simulink model "SWC_HALIN_CDD_type"  (R2021b)
settings: Solver=FixedStepDiscrete  StartTime=0.0  StopTime=10.0  FixedStep=0.005  RelTol=1e-3
undefined symbols (not defined in the file): C_TASK_5MS_S, DIDLen_APSFunConfig, DIDLen_AutoLock, DIDLen_AutoWipHSpdEN, DIDLen_DKCKey, DIDLen_DRLDis, DIDLen_DynoMode, DIDLen_FMHTimer, DIDLen_OBDReq, DIDLen_TestGroup, DIDLen_TireSize, DIDLen_USSConfig, DIDLen_WipRLSCmdCutFilter, DIDLen_WipRLSCmdHoldFilter, DIDLen_XWDMode, DIDNum_APSFunConfig, DIDNum_AutoLock, DIDNum_AutoWipHSpdEN, DIDNum_DKCKey, DIDNum_DRLDis, DIDNum_DynoMode, DIDNum_FMHTimer, DIDNum_OBDReq, DIDNum_TestGroup, DIDNum_TireSize, DIDNum_USSConfig, DIDNum_WipRLSCmdCutFilter, DIDNum_WipRLSCmdHoldFilter, DIDNum_XWDMode, ENUM_DRIVETRAIN_AWD, ENUM_DRIVETRAIN_FWD, ENUM_DRIVETRAIN_RWD, ENUM_REGENLEVEL_LV1, ENUM_REGENLEVEL_LV2, ENUM_REGENLEVEL_LV3, ENUM_REGENLEVEL_LV4, ENUM_REGENLEVEL_LV5, ENUM_REGENLEVEL_OPD, ENUM_TPMSSTA_FAT, ENUM_TPMSSTA_LOWBATTERY, ENUM_TPMSSTA_TRIGGER, FALSE, FIVE_INT, FOUR_INT, KHAL_CANBusOffDebounce_s, KHAL_DefaultRegenMode_enum, KHAL_DKCDecryptEnable_flg_ovrdflg, KHAL_DKCDecryptEnable_flg_ovrdval, KHAL_RandomNumberY1_enum, KHAL_RandomNumberY2_enum, KHAL_RandomNumberY_ovrdflg, KHAL_TPMSRESBUTT_flg_ovrdflg, KHAL_TPMSRESBUTT_flg_ovrdval, KINP_ReadVinCode_flg, ONE_INT, SIX_INT, THREE_INT, TRUE, TWO_INT, ZERO_FLOAT ... (+1)
libraries: simulink x112, hcu_lib x21, hdlsllib x15, FVT_lib x2
(part 6 of 7)

== system SWC_HALIN_CDD_type/run_SWC_HALIN_CDD_Rx_5ms_sys/Halin_CDD/Halin_SYS/RemoteControlSignal ==
  DT_CAN5_SG_TBOX1 : Inport
  CbnPreACEnaReq : Subsystem
  DrvWdwCtrlCmd : Subsystem
  PasWdwCtrlCmd : Subsystem
  PowerOffTSet : Subsystem
  RLDWdwCtrlCmd : Subsystem
  RRDWdwCtrlCmd : Subsystem
  ReDoorLock : Subsystem
  ReOutsideMirror : Subsystem
  RePwrReqTbox : Subsystem
  ReRadio : Subsystem
  RemoteACTemp : Subsystem
  RemoteAutoReq : Subsystem
  TBOXRemotePW : Subsystem
  bus_selector : BusSelector  OutputSignals=CAN5_FDC_Conn_CbnPreACEnaReq
  bus_selector1 : BusSelector  OutputSignals=CAN5_FDC_Conn_PowerOff_T_Set
  bus_selector11 : BusSelector  OutputSignals=CAN5_FDC_Conn_DrvWdwCtrl_Cmd
  bus_selector12 : BusSelector  OutputSignals=CAN5_FDC_Conn_PasWdwCtrl_Cmd
  bus_selector13 : BusSelector  OutputSignals=CAN5_FDC_Conn_RLDWdwCtrl_Cmd
  bus_selector14 : BusSelector  OutputSignals=CAN5_FDC_Conn_RRDWdwCtrl_Cmd
  bus_selector2 : BusSelector  OutputSignals=CAN5_FDC_Conn_ReOutsideMirror
  bus_selector3 : BusSelector  OutputSignals=CAN5_FDC_Conn_Re_DoorLock
  bus_selector4 : BusSelector  OutputSignals=CAN5_FDC_Conn_Re_PwrReq
  bus_selector5 : BusSelector  OutputSignals=CAN5_FDC_Conn_Re_Radio
  bus_selector6 : BusSelector  OutputSignals=CAN5_FDC_Conn_Remote_ACTemp
  bus_selector7 : BusSelector  OutputSignals=CAN5_FDC_Conn_Remote_AutoReq
  bus_selector9 : BusSelector  OutputSignals=CAN5_FDC_Conn_Remote_PW
  VHAL_CbnPreACEnaReq_enum : Outport
  VHAL_PowerOffTSet_cnt : Outport  Port=2
  VHAL_ReOutsideMirror_enum : Outport  Port=3
  VHAL_ReDoorLock_enum : Outport  Port=4
  VHAL_RePwrReqTbox_enum : Outport  Port=5
  VHAL_ReRadio_flg : Outport  Port=6
  VHAL_RemoteACTemp_C : Outport  Port=7
  VHAL_RemoteAutoReq_flg : Outport  Port=8
  VHAL_TBOXRemotePW_enum : Outport  Port=9
  VHAL_FDCConnDrvWdwCtrlCmd_pct : Outport  Port=10
  VHAL_FDCConnPasWdwCtrlCmd_pct : Outport  Port=11
  VHAL_FDCConnRLDWdwCtrlCmd_pct : Outport  Port=12
  VHAL_FDCConnRRDWdwCtrlCmd_pct : Outport  Port=13
  wires:
  DT_CAN5_SG_TBOX1/1 -> [DT_CAN5_SG_TBOX1]
  [DT_CAN5_SG_TBOX1] -> bus_selector/1
  bus_selector/1 -> CbnPreACEnaReq/1(CbnPreACEnaReq)  "<CAN5_FDC_Conn_CbnPreACEnaReq>"
  CbnPreACEnaReq/1(VHAL_CbnPreACEnaReq_enum) -> VHAL_CbnPreACEnaReq_enum/1  "VHAL_CbnPreACEnaReq_enum"
  [DT_CAN5_SG_TBOX1] -> bus_selector1/1
  bus_selector1/1 -> PowerOffTSet/1(PowerOff_T_Set)  "<CAN5_FDC_Conn_PowerOff_T_Set>"
  PowerOffTSet/1(VHAL_PowerOffTSet_cnt) -> VHAL_PowerOffTSet_cnt/1  "VHAL_PowerOffTSet_cnt"
  [DT_CAN5_SG_TBOX1] -> bus_selector2/1
  bus_selector2/1 -> ReOutsideMirror/1(ReOutsideMirror)  "<CAN5_FDC_Conn_ReOutsideMirror>"
  ReOutsideMirror/1(VHAL_ReOutsideMirror_enum) -> VHAL_ReOutsideMirror_enum/1  "VHAL_ReOutsideMirror_enum"
  [DT_CAN5_SG_TBOX1] -> bus_selector3/1
  bus_selector3/1 -> ReDoorLock/1(Re_DoorLock)  "<CAN5_FDC_Conn_Re_DoorLock>"
  ReDoorLock/1(VHAL_ReDoorLock_enum) -> VHAL_ReDoorLock_enum/1  "VHAL_ReDoorLock_enum"
  [DT_CAN5_SG_TBOX1] -> bus_selector4/1
  bus_selector4/1 -> RePwrReqTbox/1(Re_PwrReqTbox)  "<CAN5_FDC_Conn_Re_PwrReq>"
  RePwrReqTbox/1(VHAL_RePwrReqTbox_enum) -> VHAL_RePwrReqTbox_enum/1  "VHAL_RePwrReqTbox_enum"
  [DT_CAN5_SG_TBOX1] -> bus_selector5/1
  bus_selector5/1 -> ReRadio/1(Re_Radio)  "<CAN5_FDC_Conn_Re_Radio>"
  ReRadio/1(VHAL_ReRadio_flg) -> VHAL_ReRadio_flg/1  "VHAL_ReRadio_flg"
  [DT_CAN5_SG_TBOX1] -> bus_selector6/1
  bus_selector6/1 -> RemoteACTemp/1(Remote_ACTemp)  "<CAN5_FDC_Conn_Remote_ACTemp>"
  RemoteACTemp/1(VHAL_RemoteACTemp_C) -> VHAL_RemoteACTemp_C/1  "VHAL_RemoteACTemp_C"
  [DT_CAN5_SG_TBOX1] -> bus_selector7/1
  bus_selector7/1 -> RemoteAutoReq/1(Remote_AutoReq)  "<CAN5_FDC_Conn_Remote_AutoReq>"
  RemoteAutoReq/1(VHAL_RemoteAutoReq_flg) -> VHAL_RemoteAutoReq_flg/1  "VHAL_RemoteAutoReq_flg"
  [DT_CAN5_SG_TBOX1] -> bus_selector9/1
  bus_selector9/1 -> TBOXRemotePW/1(TBOX_Remote_PW)  "<CAN5_FDC_Conn_Remote_PW>"
  TBOXRemotePW/1(VHAL_TBOXRemotePW_enum) -> VHAL_TBOXRemotePW_enum/1  "VHAL_TBOXRemotePW_enum"
  [DT_CAN5_SG_TBOX1] -> bus_selector11/1
  [DT_CAN5_SG_TBOX1] -> bus_selector12/1
  [DT_CAN5_SG_TBOX1] -> bus_selector13/1
  [DT_CAN5_SG_TBOX1] -> bus_selector14/1
  bus_selector11/1 -> DrvWdwCtrlCmd/1(<CAN5_FDC_Conn_DrvWdwCtrl_Cmd>)  "<CAN5_FDC_Conn_DrvWdwCtrl_Cmd>"
  DrvWdwCtrlCmd/1(Out1) -> VHAL_FDCConnDrvWdwCtrlCmd_pct/1  "VHAL_FDCConnDrvWdwCtrlCmd_pct"
  bus_selector12/1 -> PasWdwCtrlCmd/1(<CAN5_FDC_Conn_PasWdwCtrl_Cmd>)  "<CAN5_FDC_Conn_PasWdwCtrl_Cmd>"
  PasWdwCtrlCmd/1(Out1) -> VHAL_FDCConnPasWdwCtrlCmd_pct/1  "VHAL_FDCConnPasWdwCtrlCmd_pct"
  bus_selector13/1 -> RLDWdwCtrlCmd/1(<CAN5_FDC_Conn_RLDWdwCtrl_Cmd>)  "<CAN5_FDC_Conn_RLDWdwCtrl_Cmd>"
  RLDWdwCtrlCmd/1(Out1) -> VHAL_FDCConnRLDWdwCtrlCmd_pct/1  "VHAL_FDCConnRLDWdwCtrlCmd_pct"
  bus_selector14/1 -> RRDWdwCtrlCmd/1(<CAN5_FDC_Conn_RRDWdwCtrl_Cmd>)  "<CAN5_FDC_Conn_RRDWdwCtrl_Cmd>"
  RRDWdwCtrlCmd/1(Out1) -> VHAL_FDCConnRRDWdwCtrlCmd_pct/1  "VHAL_FDCConnRRDWdwCtrlCmd_pct"

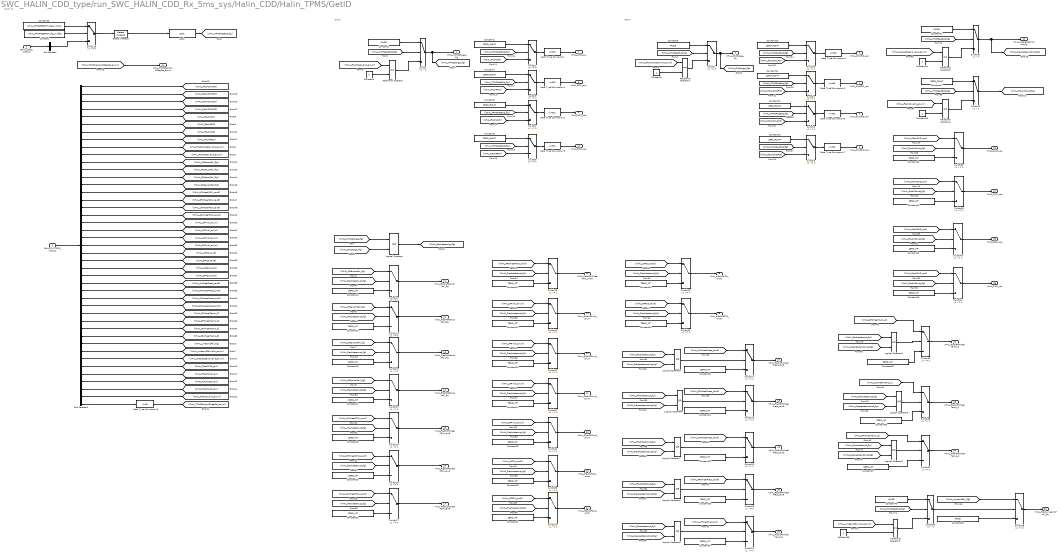
== system SWC_HALIN_CDD_type/run_SWC_HALIN_CDD_Rx_5ms_sys/Halin_CDD/Halin_TPMS/GetID ==
  note: FLASH ID
  note: GetID
  note: GetID
  BHAL_CAN2_outputs : Inport
  BHAL_SYSTPMS_outputs : Inport  Port=2
  Bus Selector : BusSelector  OutputSignals=VHAL_TPMSResButt_flg
  Bus Selector1 : BusSelector  OutputSignals=VHAL_FlashChkLFID_raw,VHAL_FlashChkRFID_raw,VHAL_FlashChkLRID_raw,VHAL_FlashChkRRID_raw,VHAL_FlashLFID_raw,VHAL_FlashRFID_raw,VHAL_FlashLRID_raw,VHAL_FlashRRID_raw,VHAL_Flashchkdatavalid_enum,VHAL_Flashdatavalid_enum,VHAL_LFSensorFail_flg,VHAL_RFSensorFail_flg,VHAL_LRSensorFail_flg,VHAL_RRSensorFail_flg,VHAL_LFWheelPSW_raw8,VHAL_RFWheelPSW_raw8,VHAL_LRWheelPSW_raw8,VHAL_RRWheelPSW_raw8,VHAL_LFPindi_enum,VHAL_RFPindi_enum,VHAL_LRPindi_enum,VHAL_RRPindi_enum,VHAL_LFP20_raw8,VHAL_RFP20_raw8,VHAL_LRP20_raw8,VHAL_RRP20_raw8,VHAL_LFWheelPress_raw8,VHAL_RFWheelPress_raw8,VHAL_LRWheelPress_raw8,VHAL_RRWheelPress_raw8,VHAL_LFWheelTemp_C,VHAL_RFWheelTemp_C,VHAL_LRWheelTemp_C,VHAL_RRWheelTemp_C,VHAL_unlearnSfali_flg,VHAL_unlearnSfailvalid_enum,VHAL_Prepresstempvalid_enum,VHAL_FlashS1ID_raw,VHAL_FlashS2ID_raw,VHAL_FlashS3ID_raw,VHAL_FlashS4ID_raw,VHAL_FlashIDvalid_enum,VHAL_TPMSSensorIDRegSta_raw
  Constant : Constant  Value=KHAL_TPMSRESBUTT_flg_ovrdflg
  Constant{1,7..13,47} (9 alike) : Constant  Value=ZERO_FLOAT
  Constant{14..37,43..46} (28 alike) : Constant  Value=ZERO_INT
  Constant{2..3,38,40..41} (5 alike) : Constant  Value=FALSE
  Constant{4..5,39,42,48} (5 alike) : Constant
  Constant6 : Constant  Value=KHAL_TPMSRESBUTT_flg_ovrdval
  Data Type Conversion{,1..7} (8 alike) : DataTypeConversion  OutDataTypeStr=uint32
  Data Type Conversion8 : DataTypeConversion  OutDataTypeStr=uint8
  Detect Increase : simulink/Logic and Bit Operations/Detect Increase  vinit=0.0  OutDataTypeStr=boolean
  Latch : hcu_lib/Basic_Blocks/Latch
  Logical Operator{,2..9} (9 alike) : Logic  Operator=OR  AllPortsSameDT=off  OutDataTypeStr=boolean
  Relational Operator{,1..4} (5 alike) : RelationalOperator  Operator===  OutDataTypeStr=boolean  RndMeth=Simplest
  Switch{,36..37,42} (4 alike) : Switch  Criteria=u2 > Threshold
  Switch{1..35,38..41} (39 alike) : Switch  Criteria=u2 ~= 0
  VHAL_TPMSStorge_flg : Outport
  VHAL_ChkStorge_flg : Outport  Port=2
  VHAL_ChkLFID_raw : Outport  Port=3
  VHAL_ChkRFID_raw : Outport  Port=4
  VHAL_ChkLRID_raw : Outport  Port=5
  VHAL_ChkRRID_raw : Outport  Port=6
  VHAL_LFID_raw : Outport  Port=7
  VHAL_RFID_raw : Outport  Port=8
  VHAL_LRID_raw : Outport  Port=9
  VHAL_RRID_raw : Outport  Port=10
  VHAL_FlashLFSensorFail_flg : Outport  Port=11
  VHAL_FlashRFSensorFail_flg : Outport  Port=12
  VHAL_FlashLRSensorFail_flg : Outport  Port=13
  VHAL_FlashRRSensorFail_flg : Outport  Port=14
  VHAL_FlashLFWheelPSW_raw8 : Outport  Port=15
  VHAL_FlashRFWheelPSW_raw8 : Outport  Port=16
  VHAL_FlashLRWheelPSW_raw8 : Outport  Port=17
  VHAL_FlashRRWheelPSW_raw8 : Outport  Port=18
  VHAL_FlashLFPindi_enum : Outport  Port=19
  VHAL_FlashRFPindi_enum : Outport  Port=20
  VHAL_FlashLRPindi_enum : Outport  Port=21
  VHAL_FlashRRPindi_enum : Outport  Port=22
  VHAL_FlashLFP20_raw8 : Outport  Port=23
  VHAL_FlashRFP20_raw8 : Outport  Port=24
  VHAL_FlashLRP20_raw8 : Outport  Port=25
  VHAL_FlashRRP20_raw8 : Outport  Port=26
  VHAL_FlashLFWheelPress_raw8 : Outport  Port=27
  VHAL_FlashRFWheelPress_raw8 : Outport  Port=28
  VHAL_FlashLRWheelPress_raw8 : Outport  Port=29
  VHAL_FlashRRWheelPress_raw8 : Outport  Port=30
  VHAL_FlashLFWheelTemp_C : Outport  Port=31
  VHAL_FlashRFWheelTemp_C : Outport  Port=32
  VHAL_FlashLRWheelTemp_C : Outport  Port=33
  VHAL_FlashRRWheelTemp_C : Outport  Port=34
  VHAL_FlashunlearnSfali_flg : Outport  Port=35
  VHAL_S1ID_raw : Outport  Port=36
  VHAL_S2ID_raw : Outport  Port=37
  VHAL_S3ID_raw : Outport  Port=38
  VHAL_S4ID_raw : Outport  Port=39
  VHAL_Prepresstemptrust_flg : Outport  Port=40
  VHAL_TPMSSensorIDRegSta_enum : Outport  Port=41
  wires:
  BHAL_CAN2_outputs/1 -> Bus Selector/1
  Latch/1 -> [VHAL_TPMSResButt_flg]
  [VHAL_TPMSResButt_flg] -> Switch4/2
  [VHAL_TPMSResButt_flg] -> Switch3/2
  [VHAL_FlashChkLFID] -> Switch6/3
  Switch3/1 -> Data Type Conversion1/1
  [VHAL_FlashRFID] -> Switch3/3
  Constant12/1 -> Switch8/1
  Constant9/1 -> Switch5/1
  [VHAL_FlashRRID] -> Switch5/3
  Constant1/1 -> Switch2/1
  Constant7/1 -> Switch3/1
  [VHAL_TPMSResButt_flg] -> Switch9/2
  [VHAL_TPMSResButt_flg] -> Switch2/2
  [VHAL_FlashLRID] -> Switch4/3
  Constant8/1 -> Switch4/1
  Switch2/1 -> Data Type Conversion/1
  [VHAL_TPMSResButt_flg] -> Switch5/2
  Switch4/1 -> Data Type Conversion2/1
  [VHAL_FlashChkLRID] -> Switch8/3
  [VHAL_FlashChkRRID] -> Switch9/3
  Constant10/1 -> Switch6/1
  Constant11/1 -> Switch7/1
  Switch8/1 -> Data Type Conversion6/1
  [VHAL_TPMSResButt_flg] -> Switch6/2
  Switch6/1 -> Data Type Conversion4/1
  Switch9/1 -> Data Type Conversion7/1
  Constant13/1 -> Switch9/1
  Switch7/1 -> Data Type Conversion5/1
  [VHAL_TPMSResButt_flg] -> Switch8/2
  [VHAL_TPMSResButt_flg] -> Switch7/2
  Switch5/1 -> Data Type Conversion3/1
  [VHAL_FlashChkRFID] -> Switch7/3
  [VHAL_FlashLFID] -> Switch2/3
  Switch10/1 -> Detect Increase/1
  Constant/1 -> Switch10/2
  Constant6/1 -> Switch10/1
  Bus Selector/1 -> Switch10/3  "<VHAL_TPMSResButt_flg>"
  [VHAL_TPMSResButt_flg] -> Switch/2
  Switch/1 -> [VHAL_TPMSStorge_flg], VHAL_TPMSStorge_flg/1
  Constant2/1 -> Switch/1
  Constant3/1 -> Switch1/1
  Switch1/1 -> [VHAL_ChkStorge_flg], VHAL_ChkStorge_flg/1
  [VHAL_TPMSResButt_flg] -> Switch1/2
  [VHAL_Flashdatavalid_enum] -> Relational Operator/1
  Relational Operator/1 -> Switch/3
  Constant4/1 -> Relational Operator/2
  Constant5/1 -> Relational Operator1/2
  Relational Operator1/1 -> Switch1/3
  [VHAL_Flashchkdatavalid_enum] -> Relational Operator1/1
  [VHAL_TPMSStorge_flg] -> Logical Operator/1
  [VHAL_ChkStorge_flg] -> Logical Operator/2
  Logical Operator/1 -> [VHAL_Flashdatatrust_flg]
  [VHAL_Flashdatatrust_flg] -> Switch11/2
  [VHAL_LFSensorFail_flg] -> Switch11/1
  Constant14/1 -> Switch11/3
  Switch11/1 -> VHAL_FlashLFSensorFail_flg/1
  Constant15/1 -> Switch12/3
  [VHAL_Flashdatatrust_flg] -> Switch12/2
  Constant16/1 -> Switch13/3
  [VHAL_Flashdatatrust_flg] -> Switch13/2
  Constant17/1 -> Switch14/3
  [VHAL_Flashdatatrust_flg] -> Switch14/2
  Constant18/1 -> Switch15/3
  [VHAL_Flashdatatrust_flg] -> Switch15/2
  Constant19/1 -> Switch16/3
  [VHAL_Flashdatatrust_flg] -> Switch16/2
  Constant20/1 -> Switch17/3
  [VHAL_Flashdatatrust_flg] -> Switch17/2
  Constant21/1 -> Switch18/3
  [VHAL_Flashdatatrust_flg] -> Switch18/2
  [VHAL_RFSensorFail_flg] -> Switch12/1
  [VHAL_LRSensorFail_flg] -> Switch13/1
  [VHAL_RRSensorFail_flg] -> Switch14/1
  [VHAL_LFWheelPSW_raw8] -> Switch15/1
  [VHAL_RFWheelPSW_raw8] -> Switch16/1
  [VHAL_LRWheelPSW_raw8] -> Switch17/1
  [VHAL_RRWheelPSW_raw8] -> Switch18/1
  Constant22/1 -> Switch19/3
  [VHAL_Flashdatatrust_flg] -> Switch19/2
  Constant23/1 -> Switch20/3
  [VHAL_Flashdatatrust_flg] -> Switch20/2
  Constant24/1 -> Switch21/3
  [VHAL_Flashdatatrust_flg] -> Switch21/2
  Constant25/1 -> Switch22/3
  [VHAL_Flashdatatrust_flg] -> Switch22/2
  [VHAL_LFPindi_enum] -> Switch19/1
  [VHAL_RFPindi_enum] -> Switch20/1
  [VHAL_LRPindi_enum] -> Switch21/1
  [VHAL_RRPindi_enum] -> Switch22/1
  Constant26/1 -> Switch23/3
  [VHAL_Flashdatatrust_flg] -> Switch23/2
  [VHAL_LFP20_raw8] -> Switch23/1
  Constant27/1 -> Switch24/3
  [VHAL_Flashdatatrust_flg] -> Switch24/2
  [VHAL_RFP20_raw8] -> Switch24/1
  Constant28/1 -> Switch25/3
  [VHAL_Flashdatatrust_flg] -> Switch25/2
  [VHAL_LRP20_raw8] -> Switch25/1
  Constant29/1 -> Switch26/3
  [VHAL_Flashdatatrust_flg] -> Switch26/2
  [VHAL_RRP20_raw8] -> Switch26/1
  Constant30/1 -> Switch27/3
  [VHAL_LFWheelPress_raw8] -> Switch27/1
  Constant31/1 -> Switch28/3
  [VHAL_RFWheelPress_raw8] -> Switch28/1
  Constant32/1 -> Switch29/3
  [VHAL_LRWheelPress_raw8] -> Switch29/1
  Constant33/1 -> Switch30/3
  [VHAL_RRWheelPress_raw8] -> Switch30/1
  Constant34/1 -> Switch31/3
  [VHAL_LFWheelTemp_C] -> Switch31/1
  Constant35/1 -> Switch32/3
  [VHAL_RFWheelTemp_C] -> Switch32/1
  Constant36/1 -> Switch33/3
  [VHAL_LRWheelTemp_C] -> Switch33/1
  Constant37/1 -> Switch34/3
  Logical Operator2/1 -> Switch34/2
  Constant38/1 -> Switch35/3
  [VHAL_unlearnSfali_flg] -> Switch35/1
  [VHAL_RRWheelTemp_C] -> Switch34/1
  Switch12/1 -> VHAL_FlashRFSensorFail_flg/1
  Switch13/1 -> VHAL_FlashLRSensorFail_flg/1
  Switch14/1 -> VHAL_FlashRRSensorFail_flg/1
  Switch15/1 -> VHAL_FlashLFWheelPSW_raw8/1
  Switch16/1 -> VHAL_FlashRFWheelPSW_raw8/1
  Switch17/1 -> VHAL_FlashLRWheelPSW_raw8/1
  Switch18/1 -> VHAL_FlashRRWheelPSW_raw8/1
  Switch19/1 -> VHAL_FlashLFPindi_enum/1
  Switch20/1 -> VHAL_FlashRFPindi_enum/1
  Switch21/1 -> VHAL_FlashLRPindi_enum/1
  Switch22/1 -> VHAL_FlashRRPindi_enum/1
  Switch23/1 -> VHAL_FlashLFP20_raw8/1
  Switch24/1 -> VHAL_FlashRFP20_raw8/1
  Switch25/1 -> VHAL_FlashLRP20_raw8/1
  Switch26/1 -> VHAL_FlashRRP20_raw8/1
  Switch27/1 -> VHAL_FlashLFWheelPress_raw8/1
  Switch28/1 -> VHAL_FlashRFWheelPress_raw8/1
  Switch29/1 -> VHAL_FlashLRWheelPress_raw8/1
  Switch30/1 -> VHAL_FlashRRWheelPress_raw8/1
  Switch31/1 -> VHAL_FlashLFWheelTemp_C/1
  Switch32/1 -> VHAL_FlashRFWheelTemp_C/1
  Switch33/1 -> VHAL_FlashLRWheelTemp_C/1
  Switch34/1 -> VHAL_FlashRRWheelTemp_C/1
  [VHAL_unlearnSfailvalid_enum] -> Relational Operator2/1
  Constant39/1 -> Relational Operator2/2
  Constant40/1 -> Switch36/1
  [VHAL_TPMSResButt_flg] -> Switch36/2
  Switch35/1 -> VHAL_FlashunlearnSfali_flg/1
  Switch36/1 -> Switch35/2
  Relational Operator2/1 -> Switch36/3
  Constant42/1 -> Relational Operator3/2
  [VHAL_TPMSResButt_flg] -> Switch37/2
  Constant41/1 -> Switch37/1
  Relational Operator3/1 -> Switch37/3
  [VHAL_Prepresstempvalid_enum] -> Relational Operator3/1
  Switch37/1 -> VHAL_Prepresstemptrust_flg/1, [VHAL_Prepresstemptrust_flg]
  [VHAL_Flashdatatrust_flg] -> Logical Operator2/1
  [VHAL_Prepresstemptrust_flg] -> Logical Operator2/2
  [VHAL_Flashdatatrust_flg] -> Logical Operator3/1
  [VHAL_Prepresstemptrust_flg] -> Logical Operator3/2
  Logical Operator3/1 -> Switch33/2
  [VHAL_Flashdatatrust_flg] -> Logical Operator4/1
  [VHAL_Prepresstemptrust_flg] -> Logical Operator4/2
  Logical Operator4/1 -> Switch32/2
  [VHAL_Flashdatatrust_flg] -> Logical Operator5/1
  [VHAL_Prepresstemptrust_flg] -> Logical Operator5/2
  Logical Operator5/1 -> Switch31/2
  [VHAL_Flashdatatrust_flg] -> Logical Operator6/1
  [VHAL_Prepresstemptrust_flg] -> Logical Operator6/2
  Logical Operator6/1 -> Switch30/2
  [VHAL_Flashdatatrust_flg] -> Logical Operator7/1
  [VHAL_Prepresstemptrust_flg] -> Logical Operator7/2
  Logical Operator7/1 -> Switch29/2
  [VHAL_Flashdatatrust_flg] -> Logical Operator8/1
  [VHAL_Prepresstemptrust_flg] -> Logical Operator8/2
  Logical Operator8/1 -> Switch28/2
  [VHAL_Flashdatatrust_flg] -> Logical Operator9/1
  [VHAL_Prepresstemptrust_flg] -> Logical Operator9/2
  Logical Operator9/1 -> Switch27/2
  Detect Increase/1 -> Latch/1
  Data Type Conversion/1 -> VHAL_LFID_raw/1
  Data Type Conversion1/1 -> VHAL_RFID_raw/1
  Data Type Conversion2/1 -> VHAL_LRID_raw/1
  Data Type Conversion3/1 -> VHAL_RRID_raw/1
  Data Type Conversion4/1 -> VHAL_ChkLFID_raw/1
  Data Type Conversion5/1 -> VHAL_ChkRFID_raw/1
  Data Type Conversion6/1 -> VHAL_ChkLRID_raw/1
  Data Type Conversion7/1 -> VHAL_ChkRRID_raw/1
  Switch42/1 -> [VHAL_FlashIDtrust_flg]
  Constant45/1 -> Switch40/3
  Constant46/1 -> Switch41/3
  Constant44/1 -> Switch39/3
  Switch39/1 -> VHAL_S2ID_raw/1
  [VHAL_FlashS3ID_raw] -> Switch40/1
  [VHAL_FlashS2ID_raw] -> Switch39/1
  [VHAL_FlashS4ID_raw] -> Switch41/1
  Constant43/1 -> Switch38/3
  [VHAL_FlashS1ID_raw] -> Switch38/1
  [VHAL_TPMSResButt_flg] -> Switch42/2
  [VHAL_FlashIDtrust_flg] -> Switch38/2
  Switch41/1 -> VHAL_S4ID_raw/1
  [VHAL_FlashIDtrust_flg] -> Switch39/2
  Constant47/1 -> Switch42/1
  Switch40/1 -> VHAL_S3ID_raw/1
  Constant48/1 -> Relational Operator4/2
  [VHAL_FlashIDtrust_flg] -> Switch41/2
  Switch38/1 -> VHAL_S1ID_raw/1
  [VHAL_FlashIDvalid_enum] -> Relational Operator4/1
  Relational Operator4/1 -> Switch42/3
  [VHAL_FlashIDtrust_flg] -> Switch40/2
  Bus Selector1/35 -> [VHAL_unlearnSfali_flg]  "<VHAL_unlearnSfali_flg>"
  Bus Selector1/4 -> [VHAL_FlashChkRRID]  "<VHAL_FlashChkRRID_raw>"
  Bus Selector1/27 -> [VHAL_LFWheelPress_raw8]  "<VHAL_LFWheelPress_raw8>"
  Bus Selector1/19 -> [VHAL_LFPindi_enum]  "<VHAL_LFPindi_enum>"
  Bus Selector1/21 -> [VHAL_LRPindi_enum]  "<VHAL_LRPindi_enum>"
  Bus Selector1/25 -> [VHAL_LRP20_raw8]  "<VHAL_LRP20_raw8>"
  Bus Selector1/33 -> [VHAL_LRWheelTemp_C]  "<VHAL_LRWheelTemp_C>"
  Bus Selector1/26 -> [VHAL_RRP20_raw8]  "<VHAL_RRP20_raw8>"
  Bus Selector1/18 -> [VHAL_RRWheelPSW_raw8]  "<VHAL_RRWheelPSW_raw8>"
  Bus Selector1/32 -> [VHAL_RFWheelTemp_C]  "<VHAL_RFWheelTemp_C>"
  Bus Selector1/29 -> [VHAL_LRWheelPress_raw8]  "<VHAL_LRWheelPress_raw8>"
  Bus Selector1/8 -> [VHAL_FlashRRID]  "<VHAL_FlashRRID_raw>"
  Bus Selector1/12 -> [VHAL_RFSensorFail_flg]  "<VHAL_RFSensorFail_flg>"
  Bus Selector1/20 -> [VHAL_RFPindi_enum]  "<VHAL_RFPindi_enum>"
  Bus Selector1/11 -> [VHAL_LFSensorFail_flg]  "<VHAL_LFSensorFail_flg>"
  Bus Selector1/24 -> [VHAL_RFP20_raw8]  "<VHAL_RFP20_raw8>"
  Bus Selector1/22 -> [VHAL_RRPindi_enum]  "<VHAL_RRPindi_enum>"
  Bus Selector1/6 -> [VHAL_FlashRFID]  "<VHAL_FlashRFID_raw>"
  Bus Selector1/3 -> [VHAL_FlashChkLRID]  "<VHAL_FlashChkLRID_raw>"
  Bus Selector1/2 -> [VHAL_FlashChkRFID]  "<VHAL_FlashChkRFID_raw>"
  Bus Selector1/37 -> [VHAL_Prepresstempvalid_enum]  "<VHAL_Prepresstempvalid_enum>"
  Bus Selector1/34 -> [VHAL_RRWheelTemp_C]  "<VHAL_RRWheelTemp_C>"
  Bus Selector1/16 -> [VHAL_RFWheelPSW_raw8]  "<VHAL_RFWheelPSW_raw8>"
  Bus Selector1/30 -> [VHAL_RRWheelPress_raw8]  "<VHAL_RRWheelPress_raw8>"
  Bus Selector1/28 -> [VHAL_RFWheelPress_raw8]  "<VHAL_RFWheelPress_raw8>"
  Bus Selector1/14 -> [VHAL_RRSensorFail_flg]  "<VHAL_RRSensorFail_flg>"
  Bus Selector1/38 -> [VHAL_FlashS1ID_raw]  "<VHAL_FlashS1ID_raw>"
  Bus Selector1/41 -> [VHAL_FlashS4ID_raw]  "<VHAL_FlashS4ID_raw>"
  Bus Selector1/10 -> [VHAL_Flashdatavalid_enum]  "<VHAL_Flashdatavalid_enum>"
  Bus Selector1/15 -> [VHAL_LFWheelPSW_raw8]  "<VHAL_LFWheelPSW_raw8>"
  Bus Selector1/5 -> [VHAL_FlashLFID]  "<VHAL_FlashLFID_raw>"
  Bus Selector1/39 -> [VHAL_FlashS2ID_raw]  "<VHAL_FlashS2ID_raw>"
  BHAL_SYSTPMS_outputs/1 -> Bus Selector1/1
  Bus Selector1/9 -> [VHAL_Flashchkdatavalid_enum]  "<VHAL_Flashchkdatavalid_enum>"
  Bus Selector1/1 -> [VHAL_FlashChkLFID]  "<VHAL_FlashChkLFID_raw>"
  Bus Selector1/7 -> [VHAL_FlashLRID]  "<VHAL_FlashLRID_raw>"
  Bus Selector1/36 -> [VHAL_unlearnSfailvalid_enum]  "<VHAL_unlearnSfailvalid_enum>"
  Bus Selector1/23 -> [VHAL_LFP20_raw8]  "<VHAL_LFP20_raw8>"
  Bus Selector1/40 -> [VHAL_FlashS3ID_raw]  "<VHAL_FlashS3ID_raw>"
  Bus Selector1/13 -> [VHAL_LRSensorFail_flg]  "<VHAL_LRSensorFail_flg>"
  Bus Selector1/42 -> [VHAL_FlashIDvalid_enum]  "<VHAL_FlashIDvalid_enum>"
  Bus Selector1/31 -> [VHAL_LFWheelTemp_C]  "<VHAL_LFWheelTemp_C>"
  Bus Selector1/17 -> [VHAL_LRWheelPSW_raw8]  "<VHAL_LRWheelPSW_raw8>"
  Bus Selector1/43 -> Data Type Conversion8/1  "<VHAL_TPMSSensorIDRegSta_raw>"
  [VHAL_TPMSSensorIDRegSta_enum] -> VHAL_TPMSSensorIDRegSta_enum/1
  Data Type Conversion8/1 -> [VHAL_TPMSSensorIDRegSta_enum]  "VHAL_TPMSSensorIDRegSta_enum"

== system SWC_HALIN_CDD_type/run_SWC_HALIN_CDD_Rx_5ms_sys/Halin_CDD/Halin_TPMS/Subsystem ==
  note: Custom State Judgement
  note: Data Output
  note: Data Valid Judge
  TPMS_DataIn_flg : Inport
  TPMS_RawData : Inport  Port=2
  Add : Sum  Inputs=++++
  Bit Shift : hdlsllib/Logic and Bit Operations/Bit Shift  mode=Shift Left Logical  N=24
  Bit Shift1 : hdlsllib/Logic and Bit Operations/Bit Shift  mode=Shift Left Logical  N=16
  Bit Shift3 : hdlsllib/Logic and Bit Operations/Bit Shift  mode=Shift Left Logical  N=8
  Bitwise NOT : simulink/Logic and Bit Operations/Bitwise Operator  logicop=NOT  UseBitMask=off  BitMask=bin2dec('11011001')  BitMaskRealWorld=Stored Integer
  CRC8_Caculation : Subsystem
  Constant1 : Constant  Value=ENUM_TPMSSTA_TRIGGER
  Constant{4,7,9..10} (4 alike) : Constant  Value=TRUE
  Constant{5..6,8,11} (4 alike) : Constant  Value=FALSE
  Constant2 : Constant  Value=ENUM_TPMSSTA_LOWBATTERY
  Constant3 : Constant  Value=ENUM_TPMSSTA_FAT
  Data Type Conversion : DataTypeConversion  OutDataTypeStr=uint32
  Data Type Conversion1 : DataTypeConversion  OutDataTypeStr=uint8
  Data Type Conversion2 : DataTypeConversion  OutDataTypeStr=uint8
  Data Type Conversion3 : DataTypeConversion  OutDataTypeStr=uint32
  Data Type Conversion4 : DataTypeConversion  OutDataTypeStr=uint32
  Demux : Demux  Outputs=9
  Demux1 : Demux  Outputs=10
  Equal{,1..4} (5 alike) : RelationalOperator  Operator===  OutDataTypeStr=boolean  RndMeth=Simplest
  Logical Operator : Logic  Inputs=3  AllPortsSameDT=off  OutDataTypeStr=boolean
  Mux : Mux  Inputs=10
  Mux1 : Mux  Inputs=8
  Switch{,1..4} (5 alike) : Switch  Criteria=u2 ~= 0
  Unit Delay : UnitDelay  SampleTime=-1  HasFrameUpgradeWarning=on
  VHAL_TPMSDataIn_flg : Outport
  VHAL_TPMSID_raw : Outport  Port=2
  VHAL_TPMSPressure_raw : Outport  Port=3
  VHAL_TPMSTemp_raw : Outport  Port=4
  VHAL_TPMSSta_enum : Outport  Port=5
  VHAL_TPMSPressureMi_raw : Outport  Port=6
  VHAL_TPMSCRC_crc : Outport  Port=7
  VHAL_TPMSCRCCalc_crc : Outport  Port=8
  VHAL_TPMSFAT_flg : Outport  Port=9
  VHAL_TPMSBattLow_flg : Outport  Port=10
  VHAL_TPMSTrigger_flg : Outport  Port=11
  wires:
  TPMS_DataIn_flg/1 -> Data Type Conversion2/1
  [TPMSData] -> Demux/1
  Bit Shift/1 -> Add/1
  Bit Shift1/1 -> Add/2
  Bit Shift3/1 -> Add/3
  Add/1 -> VHAL_TPMSID_raw/1
  Demux/5 -> [Pressure]  "Pressure"
  Demux/7 -> [Status]  "Sta"
  Demux/8 -> [PressureMirror]  "PressureMirror"
  Demux/9 -> [CRC]  "CRC"
  Demux/1 -> [ID4]  "ID4"
  Demux/2 -> [ID3]  "ID3"
  Demux/3 -> [ID2]  "ID2"
  Demux/4 -> [ID1]  "ID1"
  Demux/6 -> [Temp]  "Temp"
  [Pressure] -> Bitwise NOT/1
  Bitwise NOT/1 -> Equal/1
  [PressureMirror] -> Equal/2
  [ID4] -> Mux1/1
  [ID3] -> Mux1/2
  [ID2] -> Mux1/3
  [ID1] -> Mux1/4
  [Pressure] -> Mux1/5
  [Temp] -> Mux1/6
  [Status] -> Mux1/7
  [PressureMirror] -> Mux1/8
  Mux1/1 -> CRC8_Caculation/1(MsgData)
  [CRC] -> Equal1/2
  Equal1/1 -> Logical Operator/1
  Equal/1 -> Logical Operator/2
  Logical Operator/1 -> [DataValid_flg]
  [DataValid_flg] -> Switch/2
  Mux/1 -> Switch/1
  Switch/1 -> Unit Delay/1, Demux1/1
  Unit Delay/1 -> Switch/3
  Data Type Conversion1/1 -> [TPMSData]
  Data Type Conversion2/1 -> [Data_in]
  CRC8_Caculation/1(CRCout) -> [CRC_Calc], Equal1/1  "CRC_Calc"
  Switch1/1 -> VHAL_TPMSFAT_flg/1
  [VHAL_TPMSSta_enum] -> Equal2/1
  Constant3/1 -> Equal2/2
  Equal2/1 -> Switch1/2
  Constant4/1 -> Switch1/1
  Constant5/1 -> Switch1/3
  Constant8/1 -> Switch2/3
  [VHAL_TPMSSta_enum] -> Equal3/1
  Constant7/1 -> Switch2/1
  Switch2/1 -> VHAL_TPMSBattLow_flg/1
  Equal3/1 -> Switch2/2
  Constant2/1 -> Equal3/2
  [Data_in] -> Logical Operator/3
  [DataValid_flg] -> Switch3/2
  Switch3/1 -> VHAL_TPMSDataIn_flg/1
  Constant6/1 -> Switch3/3
  Constant9/1 -> Switch3/1
  [ID4] -> Mux/1
  [ID3] -> Mux/2
  [ID2] -> Mux/3
  [ID1] -> Mux/4
  [Pressure] -> Mux/5
  [Temp] -> Mux/6
  [Status] -> Mux/7
  [PressureMirror] -> Mux/8
  [CRC] -> Mux/9
  [CRC_Calc] -> Mux/10
  Demux1/10 -> VHAL_TPMSCRCCalc_crc/1
  Demux1/9 -> VHAL_TPMSCRC_crc/1
  Demux1/8 -> VHAL_TPMSPressureMi_raw/1
  Demux1/7 -> [VHAL_TPMSSta_enum], VHAL_TPMSSta_enum/1
  Demux1/6 -> VHAL_TPMSTemp_raw/1
  Demux1/5 -> VHAL_TPMSPressure_raw/1
  Demux1/1 -> Data Type Conversion/1
  Demux1/2 -> Data Type Conversion3/1
  Demux1/3 -> Data Type Conversion4/1
  Data Type Conversion/1 -> Bit Shift/1
  Data Type Conversion3/1 -> Bit Shift1/1
  Data Type Conversion4/1 -> Bit Shift3/1
  Demux1/4 -> Add/4
  TPMS_RawData/1 -> Data Type Conversion1/1
  Equal4/1 -> Switch4/2
  Constant10/1 -> Switch4/1
  [VHAL_TPMSSta_enum] -> Equal4/1
  Constant11/1 -> Switch4/3
  Switch4/1 -> VHAL_TPMSTrigger_flg/1
  Constant1/1 -> Equal4/2

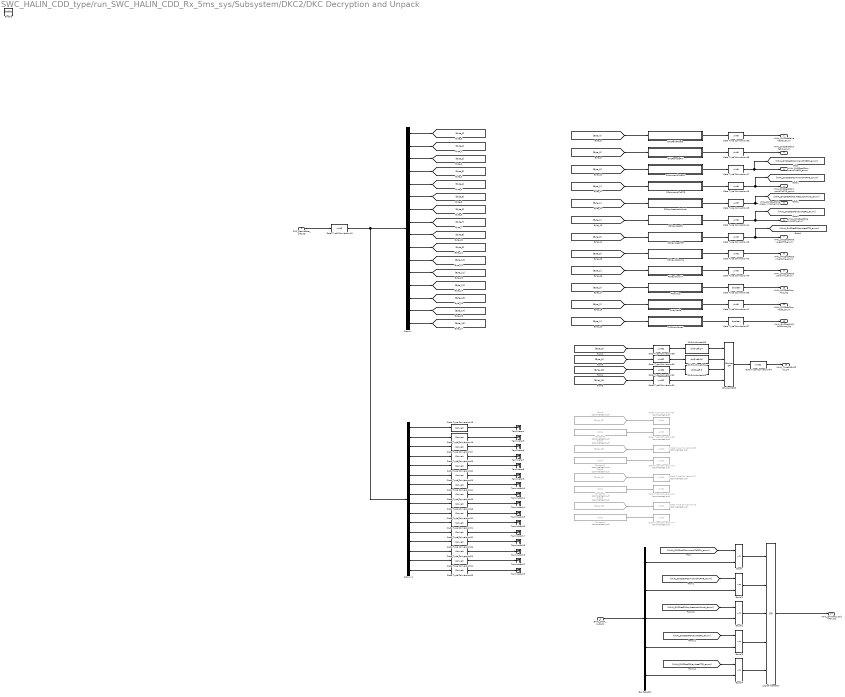
== system SWC_HALIN_CDD_type/run_SWC_HALIN_CDD_Rx_5ms_sys/Subsystem/DKC2/DKC Decryption and Unpack ==
  DKC_ResultData_16byte : Inport
  BHAL_CAN4_outputs : Inport  Port=2
  Enable : EnablePort
  Bitwise OR33 : simulink/Logic and Bit Operations/Bitwise Operator  logicop=OR  UseBitMask=off  NumInputPorts=4  BitMask=bin2dec('00000000000000000000')  BitMaskRealWorld=Stored Integer
  Bus Selector : BusSelector  OutputSignals=VHAL_PCommandToBCM_enum,VHAL_PCommandToPTG_enum,VHAL_PDKeyAreaLockUnlock_enum,VHAL_PDKeyAreaPS_enum,VHAL_PDKeyAreaPTG_enum
  Constant{1..4} (4 alike) : Constant  Commented=on  Value=0x04
  DKCReVehData : Subsystem  AncestorBlock=dkc2/DKC/Subsystem/VDKC_DKCDecryptionDATA_enum Unpack/DKCReVehData
  DKCRemotePW : Subsystem  AncestorBlock=dkc2/DKC/Subsystem/VDKC_DKCDecryptionDATA_enum Unpack/DKCRemotePW
  Data Type Conversion{16,38..47} (11 alike) : DataTypeConversion  OutDataTypeStr=uint8
  Data Type Conversion36 : DataTypeConversion  OutDataTypeStr=boolean
  Data Type Conversion37 : DataTypeConversion  OutDataTypeStr=boolean
  Data Type Conversion{48..57,59,62..66} (16 alike) : DataTypeConversion
  Data Type Conversion{58,60..61,81,94} (5 alike) : DataTypeConversion  OutDataTypeStr=uint32
  Data Type Conversion{67..74} (8 alike) : DataTypeConversion  Commented=on  OutDataTypeStr=uint8
  Demux : Demux  Outputs=16
  Demux1 : Demux  Outputs=16
  Equal{,1..4} (5 alike) : RelationalOperator  Operator=~=  OutDataTypeStr=boolean  RndMeth=Simplest
  From6 : From  Commented=on  GotoTag=Byte_12
  From7 : From  Commented=on  GotoTag=Byte_13
  From8 : From  Commented=on  GotoTag=Byte_14
  From9 : From  Commented=on  GotoTag=Byte_15
  Logical Operator : Logic  Operator=OR  Inputs=5  AllPortsSameDT=off  OutDataTypeStr=boolean
  PCommandToBCM : Subsystem  AncestorBlock=dkc2/DKC/Subsystem/VDKC_DKCDecryptionDATA_enum Unpack/PCommandToBCM
  PCommandToPTG : Subsystem  AncestorBlock=dkc2/DKC/Subsystem/VDKC_DKCDecryptionDATA_enum Unpack/PCommandToPTG
  PDKeyAreaLockUnlock : Subsystem  AncestorBlock=dkc2/DKC/Subsystem/VDKC_DKCDecryptionDATA_enum Unpack/PDKeyAreaLockUnlock
  PDKeyAreaPS : Subsystem  AncestorBlock=dkc2/DKC/Subsystem/VDKC_DKCDecryptionDATA_enum Unpack/PDKeyAreaPS
  PDKeyAreaPTG : Subsystem  AncestorBlock=dkc2/DKC/Subsystem/VDKC_DKCDecryptionDATA_enum Unpack/PDKeyAreaPTG
  PDKeyWelcome : Subsystem  AncestorBlock=dkc2/DKC/Subsystem/VDKC_DKCDecryptionDATA_enum Unpack/PDKeyWelcome
  PDkeyShowIVI : Subsystem  AncestorBlock=dkc2/DKC/Subsystem/VDKC_DKCDecryptionDATA_enum Unpack/PDkeyShowIVI
  PKeyMiss : Subsystem  AncestorBlock=dkc2/DKC/Subsystem/VDKC_DKCDecryptionDATA_enum Unpack/PKeyMiss
  PKeyMode : Subsystem  AncestorBlock=dkc2/DKC/Subsystem/VDKC_DKCDecryptionDATA_enum Unpack/PKeyMode
  PUIDLowPower : Subsystem  AncestorBlock=dkc2/DKC/Subsystem/VDKC_DKCDecryptionDATA_enum Unpack/PUIDLowPower
  Shift Arithmetic33 : ArithShift  BitShiftNumber=8  BitShiftDirection=Left
  Shift Arithmetic34 : ArithShift  BitShiftNumber=16  BitShiftDirection=Left
  Shift Arithmetic35 : ArithShift  BitShiftNumber=24  BitShiftDirection=Left
  Terminator{4..19} (16 alike) : Terminator
  VHAL_DKCDecReVehData_enum : Outport
  VHAL_DKCDecRemotePW_enum : Outport  Port=2
  VHAL_DKCDecPCommandToBCM_enum : Outport  Port=3
  VHAL_DKCDecPCommandToPTG_enum : Outport  Port=4
  VHAL_DKCDecPDKeyAreaLockUnlock_enum : Outport  Port=5
  VHAL_DKCDecPDKeyAreaPS_enum : Outport  Port=6
  VHAL_DKCDecPDKeyAreaPTG_enum : Outport  Port=7
  VHAL_DKCDecPDKeyWelcome_enum : Outport  Port=8
  VHAL_DKCDecPDkeyShowIVI_enum : Outport  Port=9
  VHAL_DKCDecPKeyMiss_flg : Outport  Port=10
  VHAL_DKCDecPKeyMode_enum : Outport  Port=11
  VHAL_DKCDecPUIDLowPower_flg : Outport  Port=12
  VHAL_TimeSNDKCFbk_cnt : Outport  Port=13
  VHAL_DKCDecryptionFail_flg : Outport  Port=14
  wires:
  Data Type Conversion53/1 -> Terminator19/1  "VHAL_DKCResultData_raw14"
  Demux1/6 -> Data Type Conversion63/1  "VHAL_DKCResultData_raw6"
  Demux1/16 -> Data Type Conversion55/1  "VHAL_DKCResultData_raw16"
  Data Type Conversion50/1 -> Terminator15/1  "VHAL_DKCResultData_raw10"
  Demux1/2 -> Data Type Conversion49/1  "VHAL_DKCResultData_raw2"
  Data Type Conversion62/1 -> Terminator8/1  "VHAL_DKCResultData_raw5"
  Data Type Conversion55/1 -> Terminator13/1  "VHAL_DKCResultData_raw16"
  Data Type Conversion49/1 -> Terminator5/1  "VHAL_DKCResultData_raw2"
  Data Type Conversion64/1 -> Terminator10/1  "VHAL_DKCResultData_raw7"
  Demux1/1 -> Data Type Conversion48/1  "VHAL_DKCResultData_raw1"
  Data Type Conversion48/1 -> Terminator4/1  "VHAL_DKCResultData_raw1"
  Data Type Conversion57/1 -> Terminator6/1  "VHAL_DKCResultData_raw3"
  Data Type Conversion56/1 -> Terminator18/1  "VHAL_DKCResultData_raw13"
  Demux1/14 -> Data Type Conversion53/1  "VHAL_DKCResultData_raw14"
  Demux1/10 -> Data Type Conversion50/1  "VHAL_DKCResultData_raw10"
  Demux1/7 -> Data Type Conversion64/1  "VHAL_DKCResultData_raw7"
  Demux1/8 -> Data Type Conversion65/1  "VHAL_DKCResultData_raw8"
  Demux1/4 -> Data Type Conversion59/1  "VHAL_DKCResultData_raw4"
  Demux1/9 -> Data Type Conversion66/1  "VHAL_DKCResultData_raw9"
  Demux1/11 -> Data Type Conversion51/1  "VHAL_DKCResultData_raw11"
  Data Type Conversion52/1 -> Terminator17/1  "VHAL_DKCResultData_raw12"
  Demux1/12 -> Data Type Conversion52/1  "VHAL_DKCResultData_raw12"
  Demux1/15 -> Data Type Conversion54/1  "VHAL_DKCResultData_raw15"
  Demux1/13 -> Data Type Conversion56/1  "VHAL_DKCResultData_raw13"
  Demux1/5 -> Data Type Conversion62/1  "VHAL_DKCResultData_raw5"
  Demux1/3 -> Data Type Conversion57/1  "VHAL_DKCResultData_raw3"
  Data Type Conversion65/1 -> Terminator11/1  "VHAL_DKCResultData_raw8"
  Data Type Conversion63/1 -> Terminator9/1  "VHAL_DKCResultData_raw6"
  Data Type Conversion54/1 -> Terminator12/1  "VHAL_DKCResultData_raw15"
  Data Type Conversion59/1 -> Terminator7/1  "VHAL_DKCResultData_raw4"
  Data Type Conversion51/1 -> Terminator16/1  "VHAL_DKCResultData_raw11"
  Data Type Conversion66/1 -> Terminator14/1  "VHAL_DKCResultData_raw9"
  PDkeyShowIVI/1(VHAL_PDkeyShowIVI_enum) -> Data Type Conversion40/1
  PDKeyAreaLockUnlock/1(VHAL_PDKeyAreaLockUnlock_enum) -> Data Type Conversion45/1
  [Byte_0] -> PDKeyWelcome/1(Byte_0)
  DKCReVehData/1(VHAL_DKCReVehData_enum) -> Data Type Conversion39/1
  [Byte_3] -> PDKeyAreaPTG/1(Byte_3)
  Demux/2 -> [Byte_1]
  PCommandToBCM/1(VHAL_PCommandToBCM_enum) -> Data Type Conversion47/1
  Data Type Conversion44/1 -> [VHAL_DKCDecPDKeyAreaPS_enum], VHAL_DKCDecPDKeyAreaPS_enum/1
  [Byte_3] -> DKCRemotePW/1(Byte_3)
  PDKeyAreaPTG/1(VHAL_PDKeyAreaPTG_enum) -> Data Type Conversion43/1
  Demux/5 -> [Byte_4]
  Demux/3 -> [Byte_2]
  PDKeyWelcome/1(VHAL_PDKeyWelcome_enum) -> Data Type Conversion42/1
  Demux/6 -> [Byte_5]
  [Byte_3] -> PKeyMiss/1(Byte_3)
  Demux/7 -> [Byte_6]
  DKCRemotePW/1(VHAL_DKCRemotePW_enum) -> Data Type Conversion38/1
  Demux/8 -> [Byte_7]
  Data Type Conversion40/1 -> VHAL_DKCDecPDkeyShowIVI_enum/1
  Demux/9 -> [Byte_8]
  Data Type Conversion42/1 -> VHAL_DKCDecPDKeyWelcome_enum/1
  Demux/10 -> [Byte_9]
  Demux/1 -> [Byte_0]
  [Byte_11] -> Data Type Conversion81/1
  Demux/11 -> [Byte_10]
  PKeyMode/1(VHAL_PKeyMode_enum) -> Data Type Conversion41/1
  Data Type Conversion43/1 -> [VHAL_DKCDecPDKeyAreaPTG_enum], VHAL_DKCDecPDKeyAreaPTG_enum/1
  Data Type Conversion94/1 -> VHAL_TimeSNDKCFbk_cnt/1
  PUIDLowPower/1(VHAL_PUIDLowPower_flg) -> Data Type Conversion37/1
  Data Type Conversion41/1 -> VHAL_DKCDecPKeyMode_enum/1
  Data Type Conversion45/1 -> [VHAL_DKCDecPDKeyAreaLockUnlock_enum], VHAL_DKCDecPDKeyAreaLockUnlock_enum/1
  [Byte_0] -> PCommandToBCM/1(Byte_0)
  PCommandToPTG/1(VHAL_PCommandToPTG_enum) -> Data Type Conversion46/1
  Data Type Conversion37/1 -> VHAL_DKCDecPUIDLowPower_flg/1
  [Byte_1] -> PDKeyAreaPS/1(Byte_1)
  [Byte_2] -> PDkeyShowIVI/1(Byte_2)
  [Byte_1] -> PDKeyAreaLockUnlock/1(Byte_1)
  Bitwise OR33/1 -> Data Type Conversion94/1
  Shift Arithmetic35/1 -> Bitwise OR33/1
  [Byte_1] -> PUIDLowPower/1(Byte_1)
  PDKeyAreaPS/1(VHAL_PDKeyAreaPS_enum) -> Data Type Conversion44/1
  Data Type Conversion58/1 -> Shift Arithmetic35/1
  Data Type Conversion60/1 -> Shift Arithmetic34/1
  Data Type Conversion46/1 -> [VHAL_DKCDecPCommandToPTG_enum], VHAL_DKCDecPCommandToPTG_enum/1
  Shift Arithmetic34/1 -> Bitwise OR33/2
  Shift Arithmetic33/1 -> Bitwise OR33/3
  Data Type Conversion36/1 -> VHAL_DKCDecPKeyMiss_flg/1
  PKeyMiss/1(VHAL_PKeyMiss_flg) -> Data Type Conversion36/1
  [Byte_8] -> Data Type Conversion58/1
  [Byte_2] -> PKeyMode/1(Byte_2)
  Data Type Conversion38/1 -> VHAL_DKCDecRemotePW_enum/1
  [Byte_4] -> DKCReVehData/1(Byte_4)
  Data Type Conversion61/1 -> Shift Arithmetic33/1
  [Byte_10] -> Data Type Conversion61/1
  [Byte_9] -> Data Type Conversion60/1
  [Byte_1] -> PCommandToPTG/1(Byte_1)
  Data Type Conversion47/1 -> [VHAL_DKCDecPCommandToBCM_enum], VHAL_DKCDecPCommandToBCM_enum/1
  Demux/12 -> [Byte_11]
  Data Type Conversion81/1 -> Bitwise OR33/4
  Data Type Conversion39/1 -> VHAL_DKCDecReVehData_enum/1
  Demux/4 -> [Byte_3]
  Data Type Conversion16/1 -> Demux/1, Demux1/1  "VHAL_DKCResultData_raw"
  DKC_ResultData_16byte/1 -> Data Type Conversion16/1
  Demux/14 -> [Byte_13]
  Demux/15 -> [Byte_14]
  Demux/16 -> [Byte_15]
  Demux/13 -> [Byte_12]
  Constant1/1 -> Data Type Conversion68/1
  Equal3/1 -> Logical Operator/4
  Constant2/1 -> Data Type Conversion70/1
  From6/1 -> Data Type Conversion67/1
  Equal1/1 -> Logical Operator/2
  Equal/1 -> Logical Operator/1
  From8/1 -> Data Type Conversion71/1
  Constant4/1 -> Data Type Conversion74/1
  Equal2/1 -> Logical Operator/3
  From9/1 -> Data Type Conversion73/1
  Constant3/1 -> Data Type Conversion72/1
  Logical Operator/1 -> VHAL_DKCDecryptionFail_flg/1
  From7/1 -> Data Type Conversion69/1
  BHAL_CAN4_outputs/1 -> Bus Selector/1
  [VHAL_DKCDecPCommandToBCM_enum] -> Equal/1
  [VHAL_DKCDecPCommandToPTG_enum] -> Equal1/1
  [VHAL_DKCDecPDKeyAreaLockUnlock_enum] -> Equal2/1
  [VHAL_DKCDecPDKeyAreaPS_enum] -> Equal3/1
  Bus Selector/1 -> Equal/2  "<VHAL_PCommandToBCM_enum>"
  Bus Selector/2 -> Equal1/2  "<VHAL_PCommandToPTG_enum>"
  Bus Selector/3 -> Equal2/2  "<VHAL_PDKeyAreaLockUnlock_enum>"
  Bus Selector/4 -> Equal3/2  "<VHAL_PDKeyAreaPS_enum>"
  [VHAL_DKCDecPDKeyAreaPTG_enum] -> Equal4/1
  Bus Selector/5 -> Equal4/2  "<VHAL_PDKeyAreaPTG_enum>"
  Equal4/1 -> Logical Operator/5

== system SWC_HALIN_CDD_type/run_SWC_HALIN_CDD_Rx_5ms_sys/Subsystem/DKC2/DKC Signal Convertor ==
  u8Array3_DKCData : Inport
  Add : Sum
  Bit Shift : hdlsllib/Logic and Bit Operations/Bit Shift  mode=Shift Right Logical  N=4
  Bit Shift1 : hdlsllib/Logic and Bit Operations/Bit Shift  mode=Shift Left Logical  N=8
  Bitwise AND : simulink/Logic and Bit Operations/Bitwise Operator  logicop=AND  UseBitMask=on  BitMask=bin2dec('00001111')  BitMaskRealWorld=Stored Integer
  Bitwise AND1 : simulink/Logic and Bit Operations/Bitwise Operator  logicop=AND  UseBitMask=on  BitMask=bin2dec('11110000')  BitMaskRealWorld=Stored Integer
  Data Type Conversion : DataTypeConversion  OutDataTypeStr=uint16
  Data Type Conversion1 : DataTypeConversion  OutDataTypeStr=uint16
  Demux : Demux  Outputs=3
  VHAL_NFCDoorSta_flg : Outport
  VHAL_NFCLidASta_flg : Outport  Port=2
  VHAL_KeyFobAreaU16_enum : Outport  Port=3
  wires:
  u8Array3_DKCData/1 -> Demux/1
  Demux/1 -> Bitwise AND1/1, Bitwise AND/1
  Bitwise AND1/1 -> Bit Shift/1
  Bitwise AND/1 -> [VHAL_NFCDoorSta_flg]
  Bit Shift/1 -> [VHAL_NFCLidASta_flg]
  [VHAL_NFCDoorSta_flg] -> VHAL_NFCDoorSta_flg/1
  [VHAL_NFCLidASta_flg] -> VHAL_NFCLidASta_flg/1
  [VHAL_KeyFobAreaU16_enum] -> VHAL_KeyFobAreaU16_enum/1
  Demux/2 -> Data Type Conversion1/1
  Add/1 -> [VHAL_KeyFobAreaU16_enum]
  Demux/3 -> Data Type Conversion/1
  Bit Shift1/1 -> Add/2
  Data Type Conversion/1 -> Bit Shift1/1
  Data Type Conversion1/1 -> Add/1

== system SWC_HALIN_CDD_type/run_SWC_HALIN_CDD_Rx_5ms_sys/Halin_CDD/Halin_SYS/RemoteControlSignal/CbnPreACEnaReq ==
  CbnPreACEnaReq : Inport
  UnitConverter : DataTypeConversion  OutDataTypeStr=uint8
  VHAL_CbnPreACEnaReq_enum : Outport
  wires:
  UnitConverter/1 -> VHAL_CbnPreACEnaReq_enum/1
  CbnPreACEnaReq/1 -> UnitConverter/1

== system SWC_HALIN_CDD_type/run_SWC_HALIN_CDD_Rx_5ms_sys/Halin_CDD/Halin_SYS/RemoteControlSignal/DrvWdwCtrlCmd ==
  <CAN5_FDC_Conn_DrvWdwCtrl_Cmd> : Inport
  Data Type Conversion : DataTypeConversion  OutDataTypeStr=uint8
  Out1 : Outport
  wires:
  Data Type Conversion/1 -> Out1/1
  <CAN5_FDC_Conn_DrvWdwCtrl_Cmd>/1 -> Data Type Conversion/1

== system SWC_HALIN_CDD_type/run_SWC_HALIN_CDD_Rx_5ms_sys/Halin_CDD/Halin_SYS/RemoteControlSignal/PasWdwCtrlCmd ==
  <CAN5_FDC_Conn_PasWdwCtrl_Cmd> : Inport
  Data Type Conversion1 : DataTypeConversion  OutDataTypeStr=uint8
  Out1 : Outport
  wires:
  <CAN5_FDC_Conn_PasWdwCtrl_Cmd>/1 -> Data Type Conversion1/1
  Data Type Conversion1/1 -> Out1/1

== system SWC_HALIN_CDD_type/run_SWC_HALIN_CDD_Rx_5ms_sys/Halin_CDD/Halin_SYS/RemoteControlSignal/PowerOffTSet ==
  PowerOff_T_Set : Inport
  UnitConverter : DataTypeConversion  OutDataTypeStr=uint8
  convert_in : FVT_lib/hal/convert_in  gain=1  offset=1
  VHAL_PowerOffTSet_cnt : Outport
  wires:
  convert_in/1 -> VHAL_PowerOffTSet_cnt/1
  UnitConverter/1 -> convert_in/1
  PowerOff_T_Set/1 -> UnitConverter/1

== system SWC_HALIN_CDD_type/run_SWC_HALIN_CDD_Rx_5ms_sys/Halin_CDD/Halin_SYS/RemoteControlSignal/RLDWdwCtrlCmd ==
  <CAN5_FDC_Conn_RLDWdwCtrl_Cmd> : Inport
  Data Type Conversion2 : DataTypeConversion  OutDataTypeStr=uint8
  Out1 : Outport
  wires:
  <CAN5_FDC_Conn_RLDWdwCtrl_Cmd>/1 -> Data Type Conversion2/1
  Data Type Conversion2/1 -> Out1/1

== system SWC_HALIN_CDD_type/run_SWC_HALIN_CDD_Rx_5ms_sys/Halin_CDD/Halin_SYS/RemoteControlSignal/RRDWdwCtrlCmd ==
  <CAN5_FDC_Conn_RRDWdwCtrl_Cmd> : Inport
  Data Type Conversion3 : DataTypeConversion  OutDataTypeStr=uint8
  Out1 : Outport
  wires:
  <CAN5_FDC_Conn_RRDWdwCtrl_Cmd>/1 -> Data Type Conversion3/1
  Data Type Conversion3/1 -> Out1/1

== system SWC_HALIN_CDD_type/run_SWC_HALIN_CDD_Rx_5ms_sys/Halin_CDD/Halin_SYS/RemoteControlSignal/ReDoorLock ==
  Re_DoorLock : Inport
  UnitConverter : DataTypeConversion  OutDataTypeStr=uint16
  VHAL_ReDoorLock_enum : Outport
  wires:
  UnitConverter/1 -> VHAL_ReDoorLock_enum/1
  Re_DoorLock/1 -> UnitConverter/1

== system SWC_HALIN_CDD_type/run_SWC_HALIN_CDD_Rx_5ms_sys/Halin_CDD/Halin_SYS/RemoteControlSignal/ReOutsideMirror ==
  ReOutsideMirror : Inport
  UnitConverter : DataTypeConversion  OutDataTypeStr=uint8
  VHAL_ReOutsideMirror_enum : Outport
  wires:
  UnitConverter/1 -> VHAL_ReOutsideMirror_enum/1
  ReOutsideMirror/1 -> UnitConverter/1

== system SWC_HALIN_CDD_type/run_SWC_HALIN_CDD_Rx_5ms_sys/Halin_CDD/Halin_SYS/RemoteControlSignal/RePwrReqTbox ==
  Re_PwrReqTbox : Inport
  UnitConverter : DataTypeConversion  OutDataTypeStr=uint8
  VHAL_RePwrReqTbox_enum : Outport
  wires:
  UnitConverter/1 -> VHAL_RePwrReqTbox_enum/1
  Re_PwrReqTbox/1 -> UnitConverter/1

== system SWC_HALIN_CDD_type/run_SWC_HALIN_CDD_Rx_5ms_sys/Halin_CDD/Halin_SYS/RemoteControlSignal/ReRadio ==
  Re_Radio : Inport
  UnitConverter : DataTypeConversion  OutDataTypeStr=uint8
  VHAL_ReRadio_flg : Outport
  wires:
  UnitConverter/1 -> VHAL_ReRadio_flg/1
  Re_Radio/1 -> UnitConverter/1

== system SWC_HALIN_CDD_type/run_SWC_HALIN_CDD_Rx_5ms_sys/Halin_CDD/Halin_SYS/RemoteControlSignal/RemoteACTemp ==
  Remote_ACTemp : Inport
  UnitConverter : DataTypeConversion  OutDataTypeStr=uint8
  convert_in : FVT_lib/hal/convert_in  gain=0.5  offset=17
  VHAL_RemoteACTemp_C : Outport
  wires:
  convert_in/1 -> VHAL_RemoteACTemp_C/1
  UnitConverter/1 -> convert_in/1
  Remote_ACTemp/1 -> UnitConverter/1

== system SWC_HALIN_CDD_type/run_SWC_HALIN_CDD_Rx_5ms_sys/Halin_CDD/Halin_SYS/RemoteControlSignal/RemoteAutoReq ==
  Remote_AutoReq : Inport
  UnitConverter : DataTypeConversion  OutDataTypeStr=uint8
  VHAL_RemoteAutoReq_flg : Outport
  wires:
  UnitConverter/1 -> VHAL_RemoteAutoReq_flg/1
  Remote_AutoReq/1 -> UnitConverter/1

== system SWC_HALIN_CDD_type/run_SWC_HALIN_CDD_Rx_5ms_sys/Halin_CDD/Halin_SYS/RemoteControlSignal/TBOXRemotePW ==
  TBOX_Remote_PW : Inport
  UnitConverter : DataTypeConversion  OutDataTypeStr=uint8
  VHAL_TBOXRemotePW_enum : Outport
  wires:
  UnitConverter/1 -> VHAL_TBOXRemotePW_enum/1
  TBOX_Remote_PW/1 -> UnitConverter/1

== system SWC_HALIN_CDD_type/run_SWC_HALIN_CDD_Rx_5ms_sys/Halin_CDD/Halin_TPMS/Subsystem/CRC8_Caculation ==
  MsgData : Inport
  Data Type Conversion1 : DataTypeConversion  OutDataTypeStr=uint16
  Data Type Conversion2 : DataTypeConversion  OutDataTypeStr=uint8
  MATLAB Function : MATLAB Function  TreatAsAtomicUnit=on
  CRCout : Outport
  wires:
  Data Type Conversion1/1 -> MATLAB Function/1(msg_raw)
  MATLAB Function/1(CRC_Out) -> Data Type Conversion2/1
  MsgData/1 -> Data Type Conversion1/1
  Data Type Conversion2/1 -> CRCout/1

== system SWC_HALIN_CDD_type/run_SWC_HALIN_CDD_Rx_5ms_sys/Subsystem/DKC2/DKC Decryption and Unpack/DKCReVehData ==
  Byte_4 : Inport
  BitwiseAND : simulink/Logic and Bit Operations/Bitwise Operator  logicop=AND  UseBitMask=off  NumInputPorts=2  BitMask=bin2dec('11011001')  BitMaskRealWorld=Stored Integer
  BitwiseOR : simulink/Logic and Bit Operations/Bitwise Operator  logicop=OR  UseBitMask=off  BitMask=bin2dec('11011001')  BitMaskRealWorld=Stored Integer
  Constant : Constant  Value=(2^4-1)
  LeftShift : ArithShift  BitShiftDirection=Left
  RightShift : ArithShift  BitShiftNumber=4  BitShiftDirection=Right
  UnitConverter : DataTypeConversion  OutDataTypeStr=uint8
  UnitConverter1 : DataTypeConversion  OutDataTypeStr=uint8
  VHAL_DKCReVehData_enum : Outport
  wires:
  BitwiseOR/1 -> RightShift/1
  RightShift/1 -> BitwiseAND/1
  UnitConverter/1 -> BitwiseAND/2
  Constant/1 -> UnitConverter/1
  BitwiseAND/1 -> VHAL_DKCReVehData_enum/1
  LeftShift/1 -> BitwiseOR/1
  UnitConverter1/1 -> LeftShift/1
  Byte_4/1 -> UnitConverter1/1

== system SWC_HALIN_CDD_type/run_SWC_HALIN_CDD_Rx_5ms_sys/Subsystem/DKC2/DKC Decryption and Unpack/DKCRemotePW ==
  Byte_3 : Inport
  BitwiseAND : simulink/Logic and Bit Operations/Bitwise Operator  logicop=AND  UseBitMask=off  NumInputPorts=2  BitMask=bin2dec('11011001')  BitMaskRealWorld=Stored Integer
  BitwiseOR : simulink/Logic and Bit Operations/Bitwise Operator  logicop=OR  UseBitMask=off  BitMask=bin2dec('11011001')  BitMaskRealWorld=Stored Integer
  Constant : Constant  Value=(2^5-1)
  LeftShift : ArithShift  BitShiftDirection=Left
  RightShift : ArithShift  BitShiftDirection=Right
  UnitConverter : DataTypeConversion  OutDataTypeStr=uint8
  UnitConverter1 : DataTypeConversion  OutDataTypeStr=uint8
  VHAL_DKCRemotePW_enum : Outport
  wires:
  BitwiseOR/1 -> RightShift/1
  RightShift/1 -> BitwiseAND/1
  UnitConverter/1 -> BitwiseAND/2
  Constant/1 -> UnitConverter/1
  BitwiseAND/1 -> VHAL_DKCRemotePW_enum/1
  LeftShift/1 -> BitwiseOR/1
  UnitConverter1/1 -> LeftShift/1
  Byte_3/1 -> UnitConverter1/1

== system SWC_HALIN_CDD_type/run_SWC_HALIN_CDD_Rx_5ms_sys/Subsystem/DKC2/DKC Decryption and Unpack/PCommandToBCM ==
  Byte_0 : Inport
  BitwiseAND : simulink/Logic and Bit Operations/Bitwise Operator  logicop=AND  UseBitMask=off  NumInputPorts=2  BitMask=bin2dec('11011001')  BitMaskRealWorld=Stored Integer
  BitwiseOR : simulink/Logic and Bit Operations/Bitwise Operator  logicop=OR  UseBitMask=off  BitMask=bin2dec('11011001')  BitMaskRealWorld=Stored Integer
  Constant : Constant  Value=(2^4-1)
  LeftShift : ArithShift  BitShiftDirection=Left
  RightShift : ArithShift  BitShiftNumber=4  BitShiftDirection=Right
  UnitConverter : DataTypeConversion  OutDataTypeStr=uint8
  UnitConverter1 : DataTypeConversion  OutDataTypeStr=uint8
  VHAL_PCommandToBCM_enum : Outport
  wires:
  BitwiseOR/1 -> RightShift/1
  RightShift/1 -> BitwiseAND/1
  UnitConverter/1 -> BitwiseAND/2
  Constant/1 -> UnitConverter/1
  BitwiseAND/1 -> VHAL_PCommandToBCM_enum/1
  LeftShift/1 -> BitwiseOR/1
  UnitConverter1/1 -> LeftShift/1
  Byte_0/1 -> UnitConverter1/1

== system SWC_HALIN_CDD_type/run_SWC_HALIN_CDD_Rx_5ms_sys/Subsystem/DKC2/DKC Decryption and Unpack/PCommandToPTG ==
  Byte_1 : Inport
  BitwiseAND : simulink/Logic and Bit Operations/Bitwise Operator  logicop=AND  UseBitMask=off  NumInputPorts=2  BitMask=bin2dec('11011001')  BitMaskRealWorld=Stored Integer
  BitwiseOR : simulink/Logic and Bit Operations/Bitwise Operator  logicop=OR  UseBitMask=off  BitMask=bin2dec('11011001')  BitMaskRealWorld=Stored Integer
  Constant : Constant  Value=(2^3-1)
  LeftShift : ArithShift  BitShiftDirection=Left
  RightShift : ArithShift  BitShiftDirection=Right
  UnitConverter : DataTypeConversion  OutDataTypeStr=uint8
  UnitConverter1 : DataTypeConversion  OutDataTypeStr=uint8
  VHAL_PCommandToPTG_enum : Outport
  wires:
  BitwiseOR/1 -> RightShift/1
  RightShift/1 -> BitwiseAND/1
  UnitConverter/1 -> BitwiseAND/2
  Constant/1 -> UnitConverter/1
  BitwiseAND/1 -> VHAL_PCommandToPTG_enum/1
  LeftShift/1 -> BitwiseOR/1
  UnitConverter1/1 -> LeftShift/1
  Byte_1/1 -> UnitConverter1/1

== system SWC_HALIN_CDD_type/run_SWC_HALIN_CDD_Rx_5ms_sys/Subsystem/DKC2/DKC Decryption and Unpack/PDKeyAreaLockUnlock ==
  Byte_1 : Inport
  BitwiseAND : simulink/Logic and Bit Operations/Bitwise Operator  logicop=AND  UseBitMask=off  NumInputPorts=2  BitMask=bin2dec('11011001')  BitMaskRealWorld=Stored Integer
  BitwiseOR : simulink/Logic and Bit Operations/Bitwise Operator  logicop=OR  UseBitMask=off  BitMask=bin2dec('11011001')  BitMaskRealWorld=Stored Integer
  Constant : Constant  Value=(2^2-1)
  LeftShift : ArithShift  BitShiftDirection=Left
  RightShift : ArithShift  BitShiftNumber=6  BitShiftDirection=Right
  UnitConverter : DataTypeConversion  OutDataTypeStr=uint8
  UnitConverter1 : DataTypeConversion  OutDataTypeStr=uint8
  VHAL_PDKeyAreaLockUnlock_enum : Outport
  wires:
  BitwiseOR/1 -> RightShift/1
  RightShift/1 -> BitwiseAND/1
  UnitConverter/1 -> BitwiseAND/2
  Constant/1 -> UnitConverter/1
  BitwiseAND/1 -> VHAL_PDKeyAreaLockUnlock_enum/1
  LeftShift/1 -> BitwiseOR/1
  UnitConverter1/1 -> LeftShift/1
  Byte_1/1 -> UnitConverter1/1

== system SWC_HALIN_CDD_type/run_SWC_HALIN_CDD_Rx_5ms_sys/Subsystem/DKC2/DKC Decryption and Unpack/PDKeyAreaPS ==
  Byte_1 : Inport
  BitwiseAND : simulink/Logic and Bit Operations/Bitwise Operator  logicop=AND  UseBitMask=off  NumInputPorts=2  BitMask=bin2dec('11011001')  BitMaskRealWorld=Stored Integer
  BitwiseOR : simulink/Logic and Bit Operations/Bitwise Operator  logicop=OR  UseBitMask=off  BitMask=bin2dec('11011001')  BitMaskRealWorld=Stored Integer
  Constant : Constant  Value=(2^2-1)
  LeftShift : ArithShift  BitShiftDirection=Left
  RightShift : ArithShift  BitShiftNumber=4  BitShiftDirection=Right
  UnitConverter : DataTypeConversion  OutDataTypeStr=uint8
  UnitConverter1 : DataTypeConversion  OutDataTypeStr=uint8
  VHAL_PDKeyAreaPS_enum : Outport
  wires:
  BitwiseOR/1 -> RightShift/1
  RightShift/1 -> BitwiseAND/1
  UnitConverter/1 -> BitwiseAND/2
  Constant/1 -> UnitConverter/1
  BitwiseAND/1 -> VHAL_PDKeyAreaPS_enum/1
  LeftShift/1 -> BitwiseOR/1
  UnitConverter1/1 -> LeftShift/1
  Byte_1/1 -> UnitConverter1/1
